simulink model "stmod_mdl"  (R2021b)
settings: Solver=ode1  StartTime=0.0  StopTime=500  FixedStep=0.001  MaxStep=0.1  MinStep=0.005  RelTol=1e-3
values from neighbouring files (symbols this model uses):
  A = [0 1; 0 0]    [pendulum_data.m]
  Am = A+B*Lx    [obsmod_data.m]    (also in outmod_data.m; outmodc_data.m; stmod_data.m = A+B*F)
  B = [0;1]    [pendulum_data.m]
  Bm = B*-inv(Cm*inv(Am)*B)    [obsmod_data.m]    (also in outmod_data.m; outmodc_data.m; stmod_data.m = B*G)
  C = C([1,3],:)    [comp_data.m]    (also in pendulum_data.m = [1 1])
  L = -inv(S*B)*(S*Am-Phi*S)    [stmod_data.m]
  rho = 1    [comp_data.m]    (also in obsint_data.m; obsmod_data.m; outmod_data.m; outmodc_data.m)
  S = rpp(A,B,psm)    [obsint_data.m]    (also in stint_data.m = [M eye(mm)]*Trtilde'; stmod_data.m = inv(S*B)*S; streg_data.m = rpp(A,B,sp))
  x0 = zeros(1,n)    [comp_data.m]    (also in obsint_data.m; obsmod_data.m; outmod_data.m; outmodc_data.m)
  xm0 = zeros(1,n)    [stmod_data.m]
undefined symbols (not defined in the file or in its folder): Lr, Lrc, m, n, P
settings Model: Creator=w.schwamm  LastModifiedBy=w.schwamm
settings DataIOCC: SaveOutput=off  SaveTime=off  ReturnWorkspaceOutputs=off  StateSaveName=x  TimeSaveName=t  OutputSaveName=y

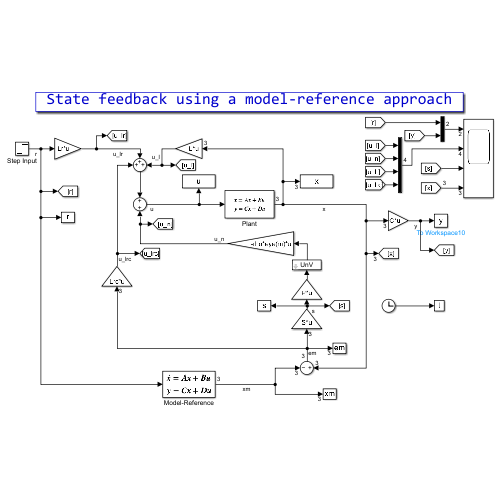
[thumbnail: Simulink's stored preview of the top-level diagram]
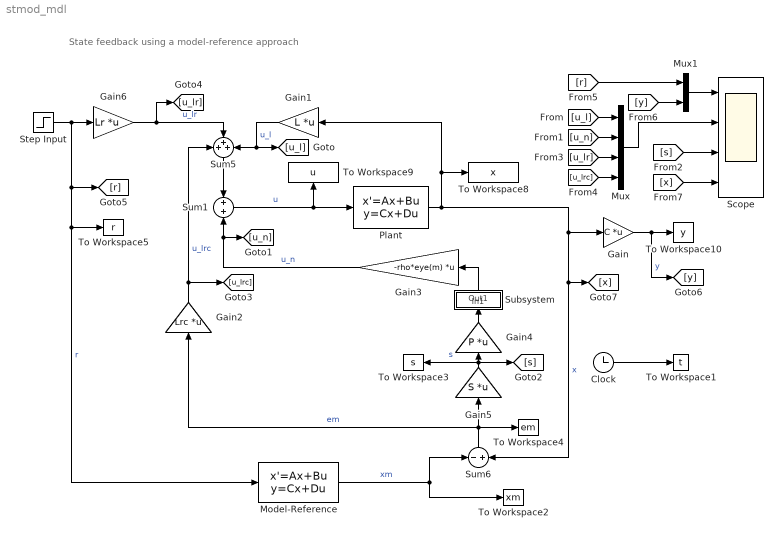
== system stmod_mdl ==
  note: State feedback using a model-reference approach
  Clock : Clock
  Gain : Gain  Gain=C  Multiplication=Matrix(K*u)
  Gain1 : Gain  Gain=L  Multiplication=Matrix(K*u)
  Gain2 : Gain  Gain=Lrc  Multiplication=Matrix(K*u)
  Gain3 : Gain  Gain=-rho*eye(m)  Multiplication=Matrix(K*u)
  Gain4 : Gain  Gain=P  Multiplication=Matrix(K*u)
  Gain5 : Gain  Gain=S  Multiplication=Matrix(K*u)
  Gain6 : Gain  Gain=Lr  Multiplication=Matrix(K*u)
  Model-Reference : StateSpace  A=Am  B=Bm  C=eye(n)  D=zeros(n,m)  InitialCondition=xm0
  Mux : Mux
  Mux1 : Mux  Inputs=2
  Plant : StateSpace  A=A  B=B  C=eye(n)  D=zeros(n,m)  InitialCondition=x0
  Scope : Scope  NumInputPorts=4
  Step Input : Step  Time=0  After=0.1  SampleTime=0
  Subsystem : Subsystem  mask{delta=0.05}
      mask prompts: delta "Unit vector delta:"
      mask Display: disp('UnV')
  Sum1 : Sum
  Sum5 : Sum  Inputs=+++
  Sum6 : Sum  Inputs=-+
  To Workspace1 : ToWorkspace  VariableName=t  SaveFormat=Timeseries  SampleTime=-1
      settings: MaxDataPoints=1000000
  To Workspace10 : ToWorkspace  VariableName=y  SaveFormat=Timeseries  SampleTime=-1
      settings: MaxDataPoints=1000000
  To Workspace2 : ToWorkspace  VariableName=xm  SaveFormat=Timeseries  SampleTime=-1
      settings: MaxDataPoints=1000000
  To Workspace3 : ToWorkspace  VariableName=s  SaveFormat=Timeseries  SampleTime=-1
      settings: MaxDataPoints=1000000
  To Workspace4 : ToWorkspace  VariableName=em  SaveFormat=Timeseries  SampleTime=-1
      settings: MaxDataPoints=1000000
  To Workspace5 : ToWorkspace  VariableName=r  SaveFormat=Timeseries  SampleTime=-1
      settings: MaxDataPoints=1000000
  To Workspace8 : ToWorkspace  VariableName=x  SaveFormat=Timeseries  SampleTime=-1
      settings: MaxDataPoints=1000000
  To Workspace9 : ToWorkspace  VariableName=u  SaveFormat=Timeseries  SampleTime=-1
      settings: MaxDataPoints=1000000
  wires:
  Clock/1 -> To Workspace1/1
  Step Input/1 -> Gain6/1, [r], To Workspace5/1, Model-Reference/1  "r"
  Subsystem/1(Out1) -> Gain3/1
  Plant/1 -> Gain1/1, To Workspace8/1, [x], Sum6/2, Gain/1  "x"
  Sum6/1 -> To Workspace4/1, Gain2/1, Gain5/1  "em"
  Gain/1 -> [y], To Workspace10/1  "y"
  Model-Reference/1 -> Sum6/1, To Workspace2/1  "xm"
  Gain4/1 -> Subsystem/1(In1)
  Gain5/1 -> Gain4/1, To Workspace3/1, [s]  "s"
  Gain3/1 -> [u_n], Sum1/2  "u_n"
  Sum1/1 -> To Workspace9/1, Plant/1  "u"
  Sum5/1 -> Sum1/1
  [u_l] -> Mux/1
  [u_n] -> Mux/2
  Mux1/1 -> Scope/1
  [s] -> Scope/3
  Gain2/1 -> [u_lrc], Sum5/1  "u_lrc"
  [u_lr] -> Mux/3
  Gain6/1 -> [u_lr], Sum5/2  "u_lr"
  Gain1/1 -> Sum5/3, [u_l]  "u_l"
  [u_lrc] -> Mux/4
  [r] -> Mux1/1
  [y] -> Mux1/2
  [x] -> Scope/4
  Mux/1 -> Scope/2

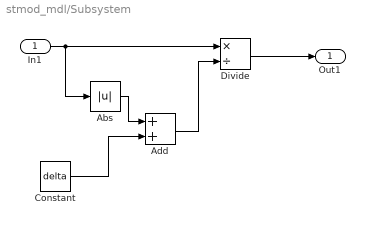
== system stmod_mdl/Subsystem ==
  In1 : Inport
  Abs : Abs
  Add : Sum
  Constant : Constant  Value=delta  SampleTime=-1
  Divide : Product  Inputs=*/
  Out1 : Outport
  wires:
  Constant/1 -> Add/2
  Add/1 -> Divide/2
  Abs/1 -> Add/1
  Divide/1 -> Out1/1
  In1/1 -> Divide/1, Abs/1
